simulink model "ECSE308_Lab_2_1_2"  (R2019b)
settings: Solver=VariableStepAuto  StartTime=0.0  StopTime=10.0  RelTol=1e-3
libraries: dsparch4 x2, commchan3 x1
settings Model: Creator=mikewang  LastModifiedBy=mikewang

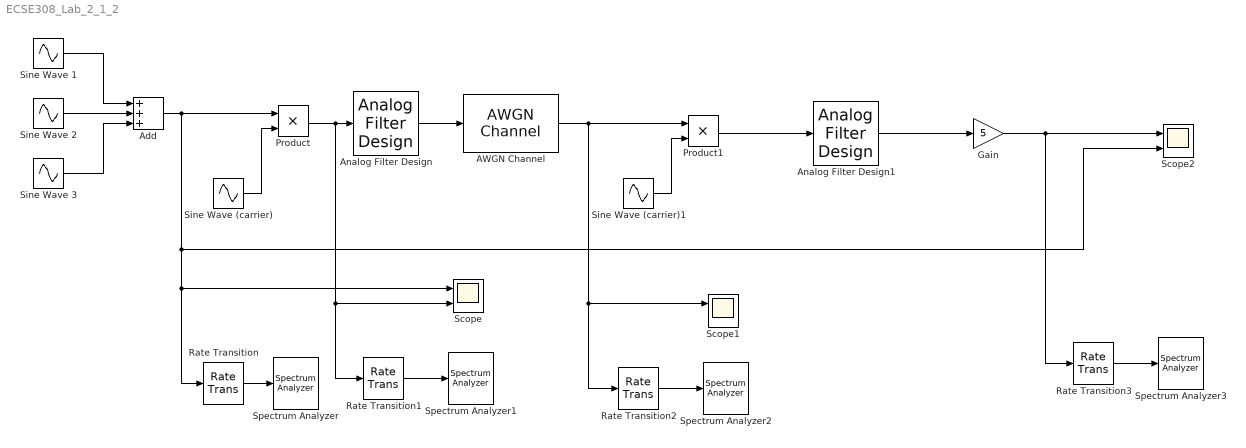
== system ECSE308_Lab_2_1_2 ==
  AWGN Channel : commchan3/AWGN Channel  InputProcessing=Columns as channels (frame based)  seed=randseed  noiseMode=Variance from mask  EbNodB=10  EsNodB=10  SNRdB=10  bitsPerSym=1  Ps=1  Tsym=1  variance=1e-3
      settings: SourceProductName=Communications Toolbox
  Add : Sum  Inputs=+++
  Analog Filter Design : dsparch4/Analog Filter Design  method=Butterworth  filttype=Bandpass  N=8  Wlo=2e4*pi  Whi=4e4*pi  Rp=2  Rs=40
  Analog Filter Design1 : dsparch4/Analog Filter Design  method=Butterworth  filttype=Lowpass  N=8  Wlo=1e4*pi  Whi=80  Rp=2  Rs=40
  Gain : Gain  Gain=5
  Product : Product
  Product1 : Product
  Rate Transition{,1..3} (4 alike) : RateTransition  OutPortSampleTime=1/50000
  Scope : Scope  NumInputPorts=2
  Scope1 : Scope  NumInputPorts=2
  Scope2 : Scope  NumInputPorts=2
  Sine Wave (carrier) : Sin  Frequency=30000*pi  Phase=pi/2  SampleTime=0
  Sine Wave (carrier)1 : Sin  Frequency=30000*pi  Phase=pi/2  SampleTime=0
  Sine Wave 1 : Sin  Amplitude=0.5  Frequency=1000*pi  SampleTime=0
  Sine Wave 2 : Sin  Amplitude=0.2  Frequency=600*pi  SampleTime=0
  Sine Wave 3 : Sin  Amplitude=0.3  Frequency=1200*pi  SampleTime=0
  Spectrum Analyzer{,1..3} (4 alike) : SpectrumAnalyzer
  wires:
  Sine Wave 2/1 -> Add/2
  Sine Wave 1/1 -> Add/1
  Sine Wave 3/1 -> Add/3
  Add/1 -> Scope2/2, Scope/1, Rate Transition/1, Product/1
  Sine Wave (carrier)/1 -> Product/2
  Rate Transition/1 -> Spectrum Analyzer/1
  Analog Filter Design/1 -> AWGN Channel/1
  Rate Transition1/1 -> Spectrum Analyzer1/1
  Product/1 -> Rate Transition1/1, Scope/2, Analog Filter Design/1
  Sine Wave (carrier)1/1 -> Product1/2
  Product1/1 -> Analog Filter Design1/1
  AWGN Channel/1 -> Scope1/1, Rate Transition2/1, Product1/1
  Rate Transition2/1 -> Spectrum Analyzer2/1
  Analog Filter Design1/1 -> Gain/1
  Gain/1 -> Rate Transition3/1, Scope2/1
  Rate Transition3/1 -> Spectrum Analyzer3/1
